simulink model "case2mod_scope"  (Simulink 7.7)
settings: Solver=FixedStepDiscrete  SolverMode=SingleTasking  StartTime=0.0  StopTime=100000  FixedStep=1  RelTol=1e-3
undefined symbols (not defined in the file): a_ratio_table
libraries: LookupModeling x38
settings Model: Creator=iris  LastModifiedBy=iris
settings DataIOCC: SaveOutput=off  SignalLogging=off  SaveTime=off
settings OptimizationCC: BlockReduction=off  ConditionallyExecuteInputs=off  InlineParams=on
settings DebuggingCC: AlgebraicLoopMsg=error  SingleTaskRateTransMsg=error
settings HardwareCC: ProdHWDeviceType=ASIC/FPGA->ASIC/FPGA

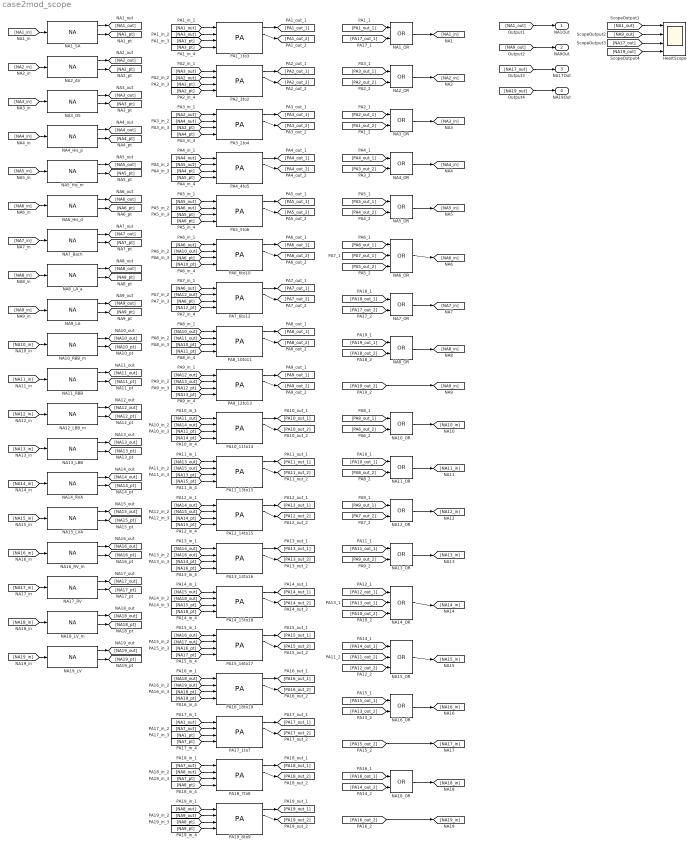
== system case2mod_scope ==
  HeartScope : Scope  NumInputPorts=4
      settings: SaveName=scopedata
  NA10_OR : Logic  Operator=OR  AllPortsSameDT=off  OutDataTypeStr=boolean
  NA10_RBB_m : LookupModeling/NA  SystemSampleTime=-1  TERP_s_m=320  TERP_defs_m=320  TRRP_s_m=120  TRRP_def_m=120  Trest_s_m=9999  Trest_def_m=9999  Terp_min_m=150  Terp_max_m=300
  NA11_OR : Logic  Operator=OR  AllPortsSameDT=off  OutDataTypeStr=boolean
  NA11_RBB : LookupModeling/NA  SystemSampleTime=-1  TERP_s_m=320  TERP_defs_m=320  TRRP_s_m=120  TRRP_def_m=120  Trest_s_m=9999  Trest_def_m=9999  Terp_min_m=150  Terp_max_m=300
  NA12_LBB_m : LookupModeling/NA  SystemSampleTime=-1  TERP_s_m=320  TERP_defs_m=320  TRRP_s_m=120  TRRP_def_m=120  Trest_s_m=9999  Trest_def_m=9999  Terp_min_m=150  Terp_max_m=300
  NA12_OR : Logic  Operator=OR  AllPortsSameDT=off  OutDataTypeStr=boolean
  NA13_LBB : LookupModeling/NA  SystemSampleTime=-1  TERP_s_m=320  TERP_defs_m=320  TRRP_s_m=120  TRRP_def_m=120  Trest_s_m=9999  Trest_def_m=9999  Terp_min_m=150  Terp_max_m=300
  NA13_OR : Logic  Operator=OR  AllPortsSameDT=off  OutDataTypeStr=boolean
  NA14_OR : Logic  Operator=OR  Inputs=3  AllPortsSameDT=off  OutDataTypeStr=boolean
  NA14_RVA : LookupModeling/NA  SystemSampleTime=-1  TERP_s_m=320  TERP_defs_m=320  TRRP_s_m=120  TRRP_def_m=120  Trest_s_m=9999  Trest_def_m=9999  Terp_min_m=150  Terp_max_m=300
  NA15_LVA : LookupModeling/NA  SystemSampleTime=-1  TERP_s_m=320  TERP_defs_m=320  TRRP_s_m=120  TRRP_def_m=120  Trest_s_m=9999  Trest_def_m=9999  Terp_min_m=150  Terp_max_m=300
  NA15_OR : Logic  Operator=OR  Inputs=3  AllPortsSameDT=off  OutDataTypeStr=boolean
  NA16_OR : Logic  Operator=OR  AllPortsSameDT=off  OutDataTypeStr=boolean
  NA16_RV_m : LookupModeling/NA  SystemSampleTime=-1  TERP_s_m=320  TERP_defs_m=320  TRRP_s_m=120  TRRP_def_m=120  Trest_s_m=9999  Trest_def_m=9999  Terp_min_m=150  Terp_max_m=300
  NA17_RV : LookupModeling/NA  SystemSampleTime=-1  TERP_s_m=320  TERP_defs_m=320  TRRP_s_m=120  TRRP_def_m=120  Trest_s_m=9999  Trest_def_m=9999  Terp_min_m=150  Terp_max_m=300
  NA18_LV_m : LookupModeling/NA  SystemSampleTime=-1  TERP_s_m=320  TERP_defs_m=320  TRRP_s_m=120  TRRP_def_m=120  Trest_s_m=9999  Trest_def_m=9999  Terp_min_m=150  Terp_max_m=300
  NA18_OR : Logic  Operator=OR  AllPortsSameDT=off  OutDataTypeStr=boolean
  NA19_LV : LookupModeling/NA  SystemSampleTime=-1  TERP_s_m=320  TERP_defs_m=320  TRRP_s_m=120  TRRP_def_m=120  Trest_s_m=9999  Trest_def_m=9999  Terp_min_m=150  Terp_max_m=300
  NA1_OR : Logic  Operator=OR  AllPortsSameDT=off  OutDataTypeStr=boolean
  NA1_SA : LookupModeling/NA  SystemSampleTime=-1  TERP_s_m=320  TERP_defs_m=320  TRRP_s_m=100  TRRP_def_m=100  Trest_s_m=800  Trest_def_m=800  Terp_min_m=150  Terp_max_m=300
  NA2_AV : LookupModeling/NA  SystemSampleTime=-1  TERP_s_m=320  TERP_defs_m=320  TRRP_s_m=350  TRRP_def_m=350  Trest_s_m=9999  Trest_def_m=9999  Terp_min_m=800  Terp_max_m=350
  NA2_OR : Logic  Operator=OR  AllPortsSameDT=off  OutDataTypeStr=boolean
  NA3_OR : Logic  Operator=OR  AllPortsSameDT=off  OutDataTypeStr=boolean
  NA3_OS : LookupModeling/NA  SystemSampleTime=-1  TERP_s_m=320  TERP_defs_m=320  TRRP_s_m=120  TRRP_def_m=120  Trest_s_m=9999  Trest_def_m=9999  Terp_min_m=150  Terp_max_m=300
  NA4_His_p : LookupModeling/NA  SystemSampleTime=-1  TERP_s_m=320  TERP_defs_m=320  TRRP_s_m=120  TRRP_def_m=120  Trest_s_m=9999  Trest_def_m=9999  Terp_min_m=150  Terp_max_m=300
  NA4_OR : Logic  Operator=OR  AllPortsSameDT=off  OutDataTypeStr=boolean
  NA5_His_m : LookupModeling/NA  SystemSampleTime=-1  TERP_s_m=320  TERP_defs_m=320  TRRP_s_m=120  TRRP_def_m=120  Trest_s_m=9999  Trest_def_m=9999  Terp_min_m=150  Terp_max_m=300
  NA5_OR : Logic  Operator=OR  AllPortsSameDT=off  OutDataTypeStr=boolean
  NA6_His_d : LookupModeling/NA  SystemSampleTime=-1  TERP_s_m=320  TERP_defs_m=320  TRRP_s_m=120  TRRP_def_m=120  Trest_s_m=9999  Trest_def_m=9999  Terp_min_m=150  Terp_max_m=300
  NA6_OR : Logic  Operator=OR  Inputs=3  AllPortsSameDT=off  OutDataTypeStr=boolean
  NA7_Bach : LookupModeling/NA  SystemSampleTime=-1  TERP_s_m=320  TERP_defs_m=320  TRRP_s_m=120  TRRP_def_m=120  Trest_s_m=9999  Trest_def_m=9999  Terp_min_m=150  Terp_max_m=300
  NA7_OR : Logic  Operator=OR  AllPortsSameDT=off  OutDataTypeStr=boolean
  NA8_LA_a : LookupModeling/NA  SystemSampleTime=-1  TERP_s_m=320  TERP_defs_m=320  TRRP_s_m=120  TRRP_def_m=120  Trest_s_m=9999  Trest_def_m=9999  Terp_min_m=150  Terp_max_m=300
  NA8_OR : Logic  Operator=OR  AllPortsSameDT=off  OutDataTypeStr=boolean
  NA9_LA : LookupModeling/NA  SystemSampleTime=-1  TERP_s_m=320  TERP_defs_m=320  TRRP_s_m=120  TRRP_def_m=120  Trest_s_m=9999  Trest_def_m=9999  Terp_min_m=150  Terp_max_m=300
  PA10_11to14 : LookupModeling/PA  SystemSampleTime=-1  min_path_par_m=9  bck_param_m=9  forw_param_m=9  a_ratio_table_m=cell2mat(a_ratio_table(10))
  PA11_13to15 : LookupModeling/PA  SystemSampleTime=-1  min_path_par_m=9  bck_param_m=10  forw_param_m=10  a_ratio_table_m=cell2mat(a_ratio_table(11))
  PA12_14to15 : LookupModeling/PA  SystemSampleTime=-1  min_path_par_m=17  bck_param_m=18  forw_param_m=18  a_ratio_table_m=cell2mat(a_ratio_table(12))
  PA13_14to16 : LookupModeling/PA  SystemSampleTime=-1  min_path_par_m=58  bck_param_m=58  forw_param_m=58  a_ratio_table_m=cell2mat(a_ratio_table(13))
  PA14_15to18 : LookupModeling/PA  SystemSampleTime=-1  min_path_par_m=46  bck_param_m=46  forw_param_m=46  a_ratio_table_m=cell2mat(a_ratio_table(14))
  PA15_16to17 : LookupModeling/PA  SystemSampleTime=-1  min_path_par_m=53  bck_param_m=53  forw_param_m=53  a_ratio_table_m=cell2mat(a_ratio_table(15))
  PA16_18to19 : LookupModeling/PA  SystemSampleTime=-1  min_path_par_m=39  bck_param_m=40  forw_param_m=40  a_ratio_table_m=cell2mat(a_ratio_table(16))
  PA17_1to7 : LookupModeling/PA  SystemSampleTime=-1  min_path_par_m=60  bck_param_m=60  forw_param_m=60  a_ratio_table_m=cell2mat(a_ratio_table(17))
  PA18_7to8 : LookupModeling/PA  SystemSampleTime=-1  min_path_par_m=34  bck_param_m=34  forw_param_m=34  a_ratio_table_m=cell2mat(a_ratio_table(18))
  PA19_8to9 : LookupModeling/PA  SystemSampleTime=-1  min_path_par_m=17  bck_param_m=18  forw_param_m=18  a_ratio_table_m=cell2mat(a_ratio_table(19))
  PA1_1to3 : LookupModeling/PA  SystemSampleTime=-1  min_path_par_m=22  bck_param_m=22  forw_param_m=22  a_ratio_table_m=cell2mat(a_ratio_table(1))
  PA2_3to2 : LookupModeling/PA  SystemSampleTime=-1  min_path_par_m=24  bck_param_m=24  forw_param_m=24  a_ratio_table_m=cell2mat(a_ratio_table(2))
  PA3_2to4 : LookupModeling/PA  SystemSampleTime=-1  min_path_par_m=93  bck_param_m=3000  forw_param_m=47  a_ratio_table_m=cell2mat(a_ratio_table(3))
  PA4_4to5 : LookupModeling/PA  SystemSampleTime=-1  min_path_par_m=16  bck_param_m=16  forw_param_m=16  a_ratio_table_m=cell2mat(a_ratio_table(4))
  PA5_5to6 : LookupModeling/PA  SystemSampleTime=-1  min_path_par_m=20  bck_param_m=20  forw_param_m=20  a_ratio_table_m=cell2mat(a_ratio_table(5))
  PA6_6to10 : LookupModeling/PA  SystemSampleTime=-1  min_path_par_m=10  bck_param_m=36  forw_param_m=36  a_ratio_table_m=cell2mat(a_ratio_table(6))
  PA7_6to12 : LookupModeling/PA  SystemSampleTime=-1  min_path_par_m=37  bck_param_m=38  forw_param_m=38  a_ratio_table_m=cell2mat(a_ratio_table(7))
  PA8_10to11 : LookupModeling/PA  SystemSampleTime=-1  min_path_par_m=10  bck_param_m=43  forw_param_m=43  a_ratio_table_m=cell2mat(a_ratio_table(8))
  PA9_12to13 : LookupModeling/PA  SystemSampleTime=-1  min_path_par_m=38  bck_param_m=38  forw_param_m=38  a_ratio_table_m=cell2mat(a_ratio_table(9))
  NA1Out : Outport
  NA9Out : Outport  Port=2
  NA17Out : Outport  Port=3
  NA19Out : Outport  Port=4
  wires:
  NA1_SA/1 -> [NA1_out]
  NA1_SA/3 -> [NA1_pt]
  [NA1_in] -> NA1_SA/1
  NA1_OR/1 -> [NA1_in]
  [PA1_out_1] -> NA1_OR/1
  [PA17_out_1] -> NA1_OR/2
  NA2_AV/1 -> [NA2_out]
  NA2_AV/3 -> [NA2_pt]
  [NA2_in] -> NA2_AV/1
  NA2_OR/1 -> [NA2_in]
  [PA3_out_1] -> NA2_OR/1
  [PA2_out_2] -> NA2_OR/2
  NA3_OS/1 -> [NA3_out]
  NA3_OS/3 -> [NA3_pt]
  [NA3_in] -> NA3_OS/1
  NA3_OR/1 -> [NA3_in]
  [PA2_out_1] -> NA3_OR/1
  [PA1_out_2] -> NA3_OR/2
  NA4_His_p/1 -> [NA4_out]
  NA4_His_p/3 -> [NA4_pt]
  [NA4_in] -> NA4_His_p/1
  NA4_OR/1 -> [NA4_in]
  [PA4_out_1] -> NA4_OR/1
  [PA3_out_2] -> NA4_OR/2
  NA5_His_m/1 -> [NA5_out]
  NA5_His_m/3 -> [NA5_pt]
  [NA5_in] -> NA5_His_m/1
  NA5_OR/1 -> [NA5_in]
  [PA5_out_1] -> NA5_OR/1
  [PA4_out_2] -> NA5_OR/2
  NA6_His_d/1 -> [NA6_out]
  NA6_His_d/3 -> [NA6_pt]
  [NA6_in] -> NA6_His_d/1
  NA6_OR/1 -> [NA6_in]
  [PA6_out_1] -> NA6_OR/1
  [PA7_out_1] -> NA6_OR/2
  [PA5_out_2] -> NA6_OR/3
  NA7_Bach/1 -> [NA7_out]
  NA7_Bach/3 -> [NA7_pt]
  [NA7_in] -> NA7_Bach/1
  NA7_OR/1 -> [NA7_in]
  [PA18_out_1] -> NA7_OR/1
  [PA17_out_2] -> NA7_OR/2
  NA8_LA_a/1 -> [NA8_out]
  NA8_LA_a/3 -> [NA8_pt]
  [NA8_in] -> NA8_LA_a/1
  NA8_OR/1 -> [NA8_in]
  [PA19_out_1] -> NA8_OR/1
  [PA18_out_2] -> NA8_OR/2
  NA9_LA/1 -> [NA9_out]
  NA9_LA/3 -> [NA9_pt]
  [NA9_in] -> NA9_LA/1
  [PA19_out_2] -> [NA9_in]
  NA10_RBB_m/1 -> [NA10_out]
  NA10_RBB_m/3 -> [NA10_pt]
  [NA10_in] -> NA10_RBB_m/1
  NA10_OR/1 -> [NA10_in]
  [PA8_out_1] -> NA10_OR/1
  [PA6_out_2] -> NA10_OR/2
  NA11_RBB/1 -> [NA11_out]
  NA11_RBB/3 -> [NA11_pt]
  [NA11_in] -> NA11_RBB/1
  NA11_OR/1 -> [NA11_in]
  [PA10_out_1] -> NA11_OR/1
  [PA8_out_2] -> NA11_OR/2
  NA12_LBB_m/1 -> [NA12_out]
  NA12_LBB_m/3 -> [NA12_pt]
  [NA12_in] -> NA12_LBB_m/1
  NA12_OR/1 -> [NA12_in]
  [PA9_out_1] -> NA12_OR/1
  [PA7_out_2] -> NA12_OR/2
  NA13_LBB/1 -> [NA13_out]
  NA13_LBB/3 -> [NA13_pt]
  [NA13_in] -> NA13_LBB/1
  NA13_OR/1 -> [NA13_in]
  [PA11_out_1] -> NA13_OR/1
  [PA9_out_2] -> NA13_OR/2
  NA14_RVA/1 -> [NA14_out]
  NA14_RVA/3 -> [NA14_pt]
  [NA14_in] -> NA14_RVA/1
  NA14_OR/1 -> [NA14_in]
  [PA12_out_1] -> NA14_OR/1
  [PA13_out_1] -> NA14_OR/2
  [PA10_out_2] -> NA14_OR/3
  NA15_LVA/1 -> [NA15_out]
  NA15_LVA/3 -> [NA15_pt]
  [NA15_in] -> NA15_LVA/1
  NA15_OR/1 -> [NA15_in]
  [PA14_out_1] -> NA15_OR/1
  [PA11_out_2] -> NA15_OR/2
  [PA12_out_2] -> NA15_OR/3
  NA16_RV_m/1 -> [NA16_out]
  NA16_RV_m/3 -> [NA16_pt]
  [NA16_in] -> NA16_RV_m/1
  NA16_OR/1 -> [NA16_in]
  [PA15_out_1] -> NA16_OR/1
  [PA13_out_2] -> NA16_OR/2
  NA17_RV/1 -> [NA17_out]
  NA17_RV/3 -> [NA17_pt]
  [NA17_in] -> NA17_RV/1
  [PA15_out_2] -> [NA17_in]
  NA18_LV_m/1 -> [NA18_out]
  NA18_LV_m/3 -> [NA18_pt]
  [NA18_in] -> NA18_LV_m/1
  NA18_OR/1 -> [NA18_in]
  [PA16_out_1] -> NA18_OR/1
  [PA14_out_2] -> NA18_OR/2
  NA19_LV/1 -> [NA19_out]
  NA19_LV/3 -> [NA19_pt]
  [NA19_in] -> NA19_LV/1
  [PA16_out_2] -> [NA19_in]
  PA1_1to3/1 -> [PA1_out_1]
  PA1_1to3/2 -> [PA1_out_2]
  [NA1_out] -> PA1_1to3/1
  [NA3_out] -> PA1_1to3/2
  [NA1_pt] -> PA1_1to3/3
  [NA3_pt] -> PA1_1to3/4
  PA2_3to2/1 -> [PA2_out_1]
  PA2_3to2/2 -> [PA2_out_2]
  [NA3_out] -> PA2_3to2/1
  [NA2_out] -> PA2_3to2/2
  [NA3_pt] -> PA2_3to2/3
  [NA2_pt] -> PA2_3to2/4
  PA3_2to4/1 -> [PA3_out_1]
  PA3_2to4/2 -> [PA3_out_2]
  [NA2_out] -> PA3_2to4/1
  [NA4_out] -> PA3_2to4/2
  [NA2_pt] -> PA3_2to4/3
  [NA4_pt] -> PA3_2to4/4
  PA4_4to5/1 -> [PA4_out_1]
  PA4_4to5/2 -> [PA4_out_2]
  [NA4_out] -> PA4_4to5/1
  [NA5_out] -> PA4_4to5/2
  [NA4_pt] -> PA4_4to5/3
  [NA5_pt] -> PA4_4to5/4
  PA5_5to6/1 -> [PA5_out_1]
  PA5_5to6/2 -> [PA5_out_2]
  [NA5_out] -> PA5_5to6/1
  [NA6_out] -> PA5_5to6/2
  [NA5_pt] -> PA5_5to6/3
  [NA6_pt] -> PA5_5to6/4
  PA6_6to10/1 -> [PA6_out_1]
  PA6_6to10/2 -> [PA6_out_2]
  [NA6_out] -> PA6_6to10/1
  [NA10_out] -> PA6_6to10/2
  [NA6_pt] -> PA6_6to10/3
  [NA10_pt] -> PA6_6to10/4
  PA7_6to12/1 -> [PA7_out_1]
  PA7_6to12/2 -> [PA7_out_2]
  [NA6_out] -> PA7_6to12/1
  [NA12_out] -> PA7_6to12/2
  [NA6_pt] -> PA7_6to12/3
  [NA12_pt] -> PA7_6to12/4
  PA8_10to11/1 -> [PA8_out_1]
  PA8_10to11/2 -> [PA8_out_2]
  [NA10_out] -> PA8_10to11/1
  [NA11_out] -> PA8_10to11/2
  [NA10_pt] -> PA8_10to11/3
  [NA11_pt] -> PA8_10to11/4
  PA9_12to13/1 -> [PA9_out_1]
  PA9_12to13/2 -> [PA9_out_2]
  [NA12_out] -> PA9_12to13/1
  [NA13_out] -> PA9_12to13/2
  [NA12_pt] -> PA9_12to13/3
  [NA13_pt] -> PA9_12to13/4
  PA10_11to14/1 -> [PA10_out_1]
  PA10_11to14/2 -> [PA10_out_2]
  [NA11_out] -> PA10_11to14/1
  [NA14_out] -> PA10_11to14/2
  [NA11_pt] -> PA10_11to14/3
  [NA14_pt] -> PA10_11to14/4
  PA11_13to15/1 -> [PA11_out_1]
  PA11_13to15/2 -> [PA11_out_2]
  [NA13_out] -> PA11_13to15/1
  [NA15_out] -> PA11_13to15/2
  [NA13_pt] -> PA11_13to15/3
  [NA15_pt] -> PA11_13to15/4
  PA12_14to15/1 -> [PA12_out_1]
  PA12_14to15/2 -> [PA12_out_2]
  [NA14_out] -> PA12_14to15/1
  [NA15_out] -> PA12_14to15/2
  [NA14_pt] -> PA12_14to15/3
  [NA15_pt] -> PA12_14to15/4
  PA13_14to16/1 -> [PA13_out_1]
  PA13_14to16/2 -> [PA13_out_2]
  [NA14_out] -> PA13_14to16/1
  [NA16_out] -> PA13_14to16/2
  [NA14_pt] -> PA13_14to16/3
  [NA16_pt] -> PA13_14to16/4
  PA14_15to18/1 -> [PA14_out_1]
  PA14_15to18/2 -> [PA14_out_2]
  [NA15_out] -> PA14_15to18/1
  [NA18_out] -> PA14_15to18/2
  [NA15_pt] -> PA14_15to18/3
  [NA18_pt] -> PA14_15to18/4
  PA15_16to17/1 -> [PA15_out_1]
  PA15_16to17/2 -> [PA15_out_2]
  [NA16_out] -> PA15_16to17/1
  [NA17_out] -> PA15_16to17/2
  [NA16_pt] -> PA15_16to17/3
  [NA17_pt] -> PA15_16to17/4
  PA16_18to19/1 -> [PA16_out_1]
  PA16_18to19/2 -> [PA16_out_2]
  [NA18_out] -> PA16_18to19/1
  [NA19_out] -> PA16_18to19/2
  [NA18_pt] -> PA16_18to19/3
  [NA19_pt] -> PA16_18to19/4
  PA17_1to7/1 -> [PA17_out_1]
  PA17_1to7/2 -> [PA17_out_2]
  [NA1_out] -> PA17_1to7/1
  [NA7_out] -> PA17_1to7/2
  [NA1_pt] -> PA17_1to7/3
  [NA7_pt] -> PA17_1to7/4
  PA18_7to8/1 -> [PA18_out_1]
  PA18_7to8/2 -> [PA18_out_2]
  [NA7_out] -> PA18_7to8/1
  [NA8_out] -> PA18_7to8/2
  [NA7_pt] -> PA18_7to8/3
  [NA8_pt] -> PA18_7to8/4
  PA19_8to9/1 -> [PA19_out_1]
  PA19_8to9/2 -> [PA19_out_2]
  [NA8_out] -> PA19_8to9/1
  [NA9_out] -> PA19_8to9/2
  [NA8_pt] -> PA19_8to9/3
  [NA9_pt] -> PA19_8to9/4
  [NA1_out] -> NA1Out/1
  [NA9_out] -> NA9Out/1
  [NA17_out] -> NA17Out/1
  [NA19_out] -> NA19Out/1
  [NA1_out] -> HeartScope/1
  [NA9_out] -> HeartScope/2
  [NA17_out] -> HeartScope/3
  [NA19_out] -> HeartScope/4
